simulink model "test_transpose"  (R2017b)
settings: Solver=FixedStepDiscrete  StartTime=0.0  StopTime=10.0  FixedStep=0.100000  RelTol=1e-3
model workspace (MAT data in the model file):
  already_pp = 1
settings Model: Creator=fconzelm  LastModifiedBy=hbourbou
settings DebuggingCC: AlgebraicLoopMsg=error  ArtificialAlgebraicLoopMsg=error  SingleTaskRateTransMsg=error

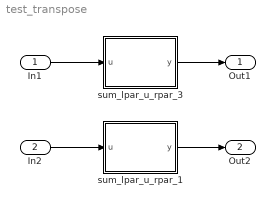
== system test_transpose ==
  In1 : Inport  PortDimensions=[1 1]
  In2 : Inport  Port=2  OutDataTypeStr=boolean  PortDimensions=[2 3]
  sum_lpar_u_rpar_1 : MATLAB Function  TreatAsAtomicUnit=on
  sum_lpar_u_rpar_3 : MATLAB Function  TreatAsAtomicUnit=on
  Out1 : Outport
  Out2 : Outport  Port=2
  wires:
  In1/1 -> sum_lpar_u_rpar_3/1(u)
  sum_lpar_u_rpar_3/1(y) -> Out1/1
  sum_lpar_u_rpar_1/1(y) -> Out2/1
  In2/1 -> sum_lpar_u_rpar_1/1(u)

== matlab function test_transpose/sum_lpar_u_rpar_1 ==
  data: u input; y output
function y = transpose1(u)

y = transpose(u);

== matlab function test_transpose/sum_lpar_u_rpar_3 ==
  data: u input; y output
function y = transpose1(u)

y = transpose(u);
